simulink subsystem "queue_populator_model"  (R2020b)
settings: Solver=VariableStepAuto  StartTime=0.0  StopTime=10.0  RelTol=1e-3
undefined symbols (not defined in the file or in its folder): kConsecutiveIndexDelta, kContainerIndexVector, kContainerLength, kFirstContainerIndex
libraries: move_index_lib x1
settings Model: Creator=rsub  LastModifiedBy=rsub

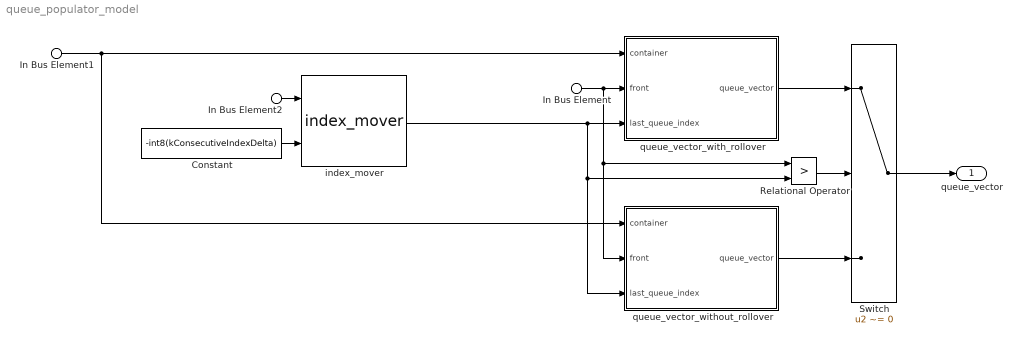
== system queue_populator_model ==
  In Bus Element : Inport  PortName=update_func_tx_bus  Element=front_index
  In Bus Element1 : Inport  PortName=update_func_tx_bus  Element=container_vector
  In Bus Element2 : Inport  PortName=update_func_tx_bus  Element=back_index
  Constant : Constant  Value=-int8(kConsecutiveIndexDelta)
  Relational Operator : RelationalOperator  Operator=>  OutDataTypeStr=boolean  RndMeth=Simplest
  Switch : Switch  Criteria=u2 ~= 0  AllowDiffInputSizes=on
  index_mover : move_index_lib/index_mover  SystemSampleTime=-1  VariantActivationTime=update diagram  Latency=0  AutoFrameSizeCalculation=off
  queue_vector_with_rollover : Subsystem
  queue_vector_without_rollover : Subsystem
  queue_vector : Outport
  wires:
  Switch/1 -> queue_vector/1
  queue_vector_with_rollover/1(queue_vector) -> Switch/1
  index_mover/1 -> queue_vector_with_rollover/3(last_queue_index), Relational Operator/2, queue_vector_without_rollover/3(last_queue_index)
  In Bus Element/1 -> queue_vector_with_rollover/2(front), Relational Operator/1, queue_vector_without_rollover/2(front)
  In Bus Element1/1 -> queue_vector_without_rollover/1(container), queue_vector_with_rollover/1(container)
  Relational Operator/1 -> Switch/2
  queue_vector_without_rollover/1(queue_vector) -> Switch/3
  In Bus Element2/1 -> index_mover/1
  Constant/1 -> index_mover/2

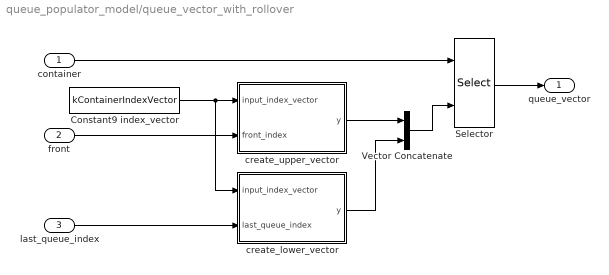
== system queue_populator_model/queue_vector_with_rollover ==
  container : Inport
  front : Inport  Port=2
  last_queue_index : Inport  Port=3
  Constant9 index_vector : Constant  Value=kContainerIndexVector
  Selector : Selector  IndexMode=Zero-based  InputPortWidth=kContainerLength  IndexOptions=Index vector (port)  Indices=[1 3]  OutputSizes=1
      settings: AttributesFormatString=%<IndexOptions>
  Vector Concatenate : Concatenate
  create_lower_vector : Subsystem
  create_upper_vector : Subsystem
  queue_vector : Outport
  wires:
  create_lower_vector/1(y) -> Vector Concatenate/2
  create_upper_vector/1(y) -> Vector Concatenate/1
  last_queue_index/1 -> create_lower_vector/2(last_queue_index)
  front/1 -> create_upper_vector/2(front_index)
  Constant9 index_vector/1 -> create_upper_vector/1(input_index_vector), create_lower_vector/1(input_index_vector)
  Vector Concatenate/1 -> Selector/2
  container/1 -> Selector/1
  Selector/1 -> queue_vector/1

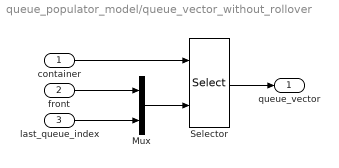
== system queue_populator_model/queue_vector_without_rollover ==
  container : Inport
  front : Inport  Port=2
  last_queue_index : Inport  Port=3
  Mux : Mux  Inputs=2
  Selector : Selector  IndexMode=Zero-based  InputPortWidth=kContainerLength  IndexOptions=Starting and ending indices (port)  Indices=[1 3]  OutputSizes=1
      settings: AttributesFormatString=%<IndexOptions>
  queue_vector : Outport
  wires:
  Mux/1 -> Selector/2
  last_queue_index/1 -> Mux/2
  container/1 -> Selector/1
  front/1 -> Mux/1
  Selector/1 -> queue_vector/1

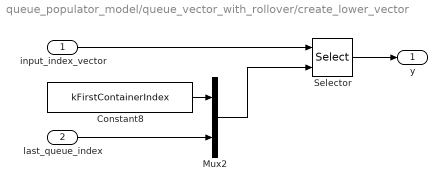
== system queue_populator_model/queue_vector_with_rollover/create_lower_vector ==
  input_index_vector : Inport
  last_queue_index : Inport  Port=2
  Constant8 : Constant  Value=kFirstContainerIndex
  Mux2 : Mux  Inputs=2
  Selector : Selector  IndexMode=Zero-based  InputPortWidth=kContainerLength  IndexOptions=Starting and ending indices (port)  Indices=[1 3]  OutputSizes=1
      settings: AttributesFormatString=%<IndexOptions>
  y : Outport
  wires:
  last_queue_index/1 -> Mux2/2
  Mux2/1 -> Selector/2
  Constant8/1 -> Mux2/1
  Selector/1 -> y/1
  input_index_vector/1 -> Selector/1

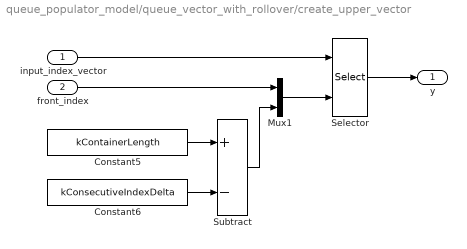
== system queue_populator_model/queue_vector_with_rollover/create_upper_vector ==
  input_index_vector : Inport
  front_index : Inport  Port=2
  Constant5 : Constant  Value=kContainerLength
  Constant6 : Constant  Value=kConsecutiveIndexDelta
  Mux1 : Mux  Inputs=2
  Selector : Selector  IndexMode=Zero-based  InputPortWidth=kContainerLength  IndexOptions=Starting and ending indices (port)  Indices=[1 3]  OutputSizes=1
      settings: AttributesFormatString=%<IndexOptions>
  Subtract : Sum  Inputs=+-
  y : Outport
  wires:
  Subtract/1 -> Mux1/2
  Mux1/1 -> Selector/2
  front_index/1 -> Mux1/1
  Constant5/1 -> Subtract/1
  Constant6/1 -> Subtract/2
  Selector/1 -> y/1
  input_index_vector/1 -> Selector/1
